simulink model "RoboticFish_Maneuverability_model"  (R2022b)
settings: Solver=ode4  StartTime=0.0  StopTime=50  FixedStep=0.01  RelTol=1e-3  EnableMultiTasking=on
libraries: sharedutil x15, matrix_library x1, dspvision x1, vrlib x1
(part 2 of 3)

== system RoboticFish_Maneuverability_model/Robotic-Fish Model & PropulsionSystem/RF Dynamics and Kinematics (Attitude rappresentation: Quaternions)/6 DOF transformation ==
  note: p q r
  note: u v w
  note: e=[eta;e1;e2;e3]
  note: eta1dot
  note: eta2dot
  eta_E : Inport
  nu : Inport  Port=2
  E1(e) : Subsystem
  E2(e) : Subsystem
  Mux : Mux  Inputs=2
  Product : Product  Inputs=**  Multiplication=Matrix(*)  SaturateOnIntegerOverflow=on  OutDataTypeStr=Inherit: Same as first input
  Product1 : Product  Inputs=**  Multiplication=Matrix(*)  SaturateOnIntegerOverflow=on  OutDataTypeStr=Inherit: Same as first input
  Selector : Selector  InputPortWidth=7  IndexOptions=Index vector (dialog)  Indices=[4 5 6 7]  OutputSizes=1
  Selector1 : Selector  InputPortWidth=6  IndexOptions=Index vector (dialog)  Indices=[1 2 3]  OutputSizes=1
  Selector2 : Selector  InputPortWidth=6  IndexOptions=Index vector (dialog)  Indices=[4 5 6]  OutputSizes=1
  etadot = J(eta_E)*nu : Outport  VectorParamsAs1DForOutWhenUnconnected=off
  E1 : Outport  Port=2  VectorParamsAs1DForOutWhenUnconnected=off
  wires:
  Product1/1 -> Mux/2
  Mux/1 -> etadot = J(eta_E)*nu/1
  Product/1 -> Mux/1
  E2(e)/1(E2) -> Product1/1
  Selector2/1 -> Product1/2
  Selector1/1 -> Product/2
  nu/1 -> Selector2/1, Selector1/1
  E1(e)/1(E1) -> Product/1, E1/1
  eta_E/1 -> Selector/1
  Selector/1 -> E1(e)/1(e), E2(e)/1(e)

== system RoboticFish_Maneuverability_model/Robotic-Fish Model & PropulsionSystem/RF Dynamics and Kinematics (Attitude rappresentation: Quaternions)/Added Mass Coriolis and centripetal matrix ==
  nu_r_B : Inport
  Gain1 : Gain  Gain=-1  SaturateOnIntegerOverflow=on  OutDataTypeStr=Inherit: Same as input  ParamDataTypeStr=Inherit: Same as input
  Gain2 : Gain  Gain=-1  SaturateOnIntegerOverflow=on  OutDataTypeStr=Inherit: Same as input  ParamDataTypeStr=Inherit: Same as input
  M11 : Constant  Value=M11
  M12 : Constant  Value=M12
  M21 : Constant  Value=M21
  M22 : Constant  Value=M22
  Matrix Concatenation : Concatenate  Mode=Multidimensional array
  Matrix Concatenation1 : Concatenate  Mode=Multidimensional array
  Matrix Concatenation2 : Concatenate  Mode=Multidimensional array  ConcatenateDimension=2
  Matrix Multiply{1..4} (4 alike) : Product  Multiplication=Matrix(*)
  Selector1 : Selector  InputPortWidth=6  IndexOptions=Index vector (dialog)  Indices=[1 2 3]  OutputSizes=1
  Selector2 : Selector  InputPortWidth=6  IndexOptions=Index vector (dialog)  Indices=[4 5 6]  OutputSizes=1
  Skew Symmetrical Operator : Subsystem
  "Skew Symmetrical Operator " : Subsystem
  Sum2 : Sum  Inputs=|++  SaturateOnIntegerOverflow=on
  Sum3 : Sum  Inputs=|++  SaturateOnIntegerOverflow=on
  Zero matrix (3 x 3) : Constant  Value=zeros(3,3)
  CA : Outport  VectorParamsAs1DForOutWhenUnconnected=off
  wires:
  Zero matrix (3 x 3)/1 -> Matrix Concatenation/1  "CA(1,1)"
  Matrix Concatenation/1 -> Matrix Concatenation2/1
  Matrix Concatenation1/1 -> Matrix Concatenation2/2
  Matrix Multiply2/1 -> Sum2/1  "M11 * nu_r1_B"
  Matrix Multiply1/1 -> Sum2/2  "M12 * nu_r2_B"
  Matrix Multiply3/1 -> Sum3/1  "M21 * nu_r1_B"
  Selector1/1 -> Matrix Multiply2/2, Matrix Multiply3/2  "nu_r1_B"
  Matrix Multiply4/1 -> Sum3/2  "M22 * nu_r2_B"
  Selector2/1 -> Matrix Multiply1/2, Matrix Multiply4/2  "nu_r2_B"
  Sum2/1 -> "Skew Symmetrical Operator "/1(v)
  Sum3/1 -> Skew Symmetrical Operator/1(v)
  "Skew Symmetrical Operator "/1(S(V)) -> Gain1/1
  Skew Symmetrical Operator/1(S(V)) -> Gain2/1
  Gain1/1 -> Matrix Concatenation1/1, Matrix Concatenation/2  "CA(1,2)"
  Gain2/1 -> Matrix Concatenation1/2  "CA(2,2)"
  nu_r_B/1 -> Selector1/1, Selector2/1
  Matrix Concatenation2/1 -> CA/1
  M11/1 -> Matrix Multiply2/1
  M12/1 -> Matrix Multiply1/1
  M21/1 -> Matrix Multiply3/1
  M22/1 -> Matrix Multiply4/1

== system RoboticFish_Maneuverability_model/Robotic-Fish Model & PropulsionSystem/RF Dynamics and Kinematics (Attitude rappresentation: Quaternions)/Damping forces ==
  nu_r_B : Inport
  Abs : Abs
  Create Diagonal Matrix : matrix_library/Create Diagonal Matrix
  Gain : Gain  Gain=-1
  Linear Damping Matrix : Constant  Value=DL
  Matrix Multiply : Product  Multiplication=Matrix(*)
  Product : Product  SaturateOnIntegerOverflow=on  OutDataTypeStr=Inherit: Same as first input
  Quadratic Damping Vector : Constant  Value=dQ
  Reshape1 : Reshape  OutputDimensionality=Column vector (2-D)
  Reshape2 : Reshape  OutputDimensionality=Column vector (2-D)  OutputDimensions=[6,6]
  Sum1 : Sum  Inputs=|++  SaturateOnIntegerOverflow=on
  D * nu_B : Outport  VectorParamsAs1DForOutWhenUnconnected=off
  wires:
  Reshape2/1 -> Product/1
  Reshape1/1 -> Matrix Multiply/2, Abs/1
  nu_r_B/1 -> Reshape1/1
  Linear Damping Matrix/1 -> Sum1/1
  Create Diagonal Matrix/1 -> Sum1/2
  Product/1 -> Create Diagonal Matrix/1
  Abs/1 -> Product/2  "abs(nu_B)"
  Quadratic Damping Vector/1 -> Reshape2/1  "dQ"
  Matrix Multiply/1 -> D * nu_B/1
  Sum1/1 -> Gain/1  "D"
  Gain/1 -> Matrix Multiply/1

== system RoboticFish_Maneuverability_model/Robotic-Fish Model & PropulsionSystem/RF Dynamics and Kinematics (Attitude rappresentation: Quaternions)/Quaternion normalisation ==
  eta_E : Inport
  Mux : Mux  Inputs=2
  Product : Product  Inputs=*/  SaturateOnIntegerOverflow=on  OutDataTypeStr=Inherit: Same as first input
  Reshape : Reshape  OutputDimensionality=Column vector (2-D)
  Selector : Selector  InputPortWidth=7  IndexOptions=Index vector (dialog)  Indices=[1 2 3]  OutputSizes=1
  Selector1 : Selector  InputPortWidth=7  IndexOptions=Index vector (dialog)  Indices=[4 5 6 7]  OutputSizes=1
  norm 1x4 vector : Subsystem
  eta_E (norm) : Outport  VectorParamsAs1DForOutWhenUnconnected=off
  wires:
  eta_E/1 -> Selector1/1, Selector/1  "eta_E"
  Selector1/1 -> norm 1x4 vector/1(Inport), Product/1
  Selector/1 -> Mux/1
  Product/1 -> Mux/2
  Mux/1 -> Reshape/1
  Reshape/1 -> eta_E (norm)/1
  norm 1x4 vector/1(norm) -> Product/2

== system RoboticFish_Maneuverability_model/Robotic-Fish Model & PropulsionSystem/RF Dynamics and Kinematics (Attitude rappresentation: Quaternions)/Restoring forces ==
  eta_E : Inport
  3x3 Cross Product : sharedutil/3x3 Cross Product  aMode=aMode
  3x3 Cross Product1 : sharedutil/3x3 Cross Product  aMode=aMode
  E1(e) : Subsystem
  Gain : Gain  Gain=-1  SaturateOnIntegerOverflow=on  OutDataTypeStr=Inherit: Same as input  ParamDataTypeStr=Inherit: Same as input
  Matrix Multiply : Product  Multiplication=Matrix(*)
  Matrix Multiply1 : Product  Multiplication=Matrix(*)
  Mux : Mux  Inputs=2
  Selector : Selector  InputPortWidth=7  IndexOptions=Index vector (dialog)  Indices=[4 5 6 7]  OutputSizes=1
  Sum1 : Sum  Inputs=|++  SaturateOnIntegerOverflow=on
  Sum2 : Sum  Inputs=|++  SaturateOnIntegerOverflow=on
  Transpose : Math  Operator=transpose  SignedPower=on
  fB_E : Constant  Value=[0;0;-B]
  fG_E : Constant  Value=[0;0;W]
  rB_B : Constant  Value=rB_B
  rG_B : Constant  Value=rG_B
  g(eta_E)_B : Outport  VectorParamsAs1DForOutWhenUnconnected=off
  wires:
  E1(e)/1(E1) -> Transpose/1  "E1(e)"
  Transpose/1 -> Matrix Multiply/1, Matrix Multiply1/1  "E1(e)^T"
  fG_E/1 -> Matrix Multiply/2
  fB_E/1 -> Matrix Multiply1/2
  Matrix Multiply/1 -> Sum1/1, 3x3 Cross Product/2  "fG_B"
  Matrix Multiply1/1 -> Sum1/2, 3x3 Cross Product1/2  "fB_B"
  rG_B/1 -> 3x3 Cross Product/1
  Sum1/1 -> Mux/1  "fG_B + fB_B"
  3x3 Cross Product/1 -> Sum2/1  "rG_B x fG_B"
  3x3 Cross Product1/1 -> Sum2/2  "rG_B x fG_B"
  rB_B/1 -> 3x3 Cross Product1/1
  Sum2/1 -> Mux/2
  Mux/1 -> Gain/1
  Gain/1 -> g(eta_E)_B/1
  Selector/1 -> E1(e)/1(e)  "e"
  eta_E/1 -> Selector/1  "E1(e)"

== system RoboticFish_Maneuverability_model/Robotic-Fish Model & PropulsionSystem/RF Dynamics and Kinematics (Attitude rappresentation: Quaternions)/Rigid-body Coriolis and centripetal matrix ==
  nu_B : Inport
  Gain : Gain  Gain=m  SaturateOnIntegerOverflow=on  OutDataTypeStr=Inherit: Same as input  ParamDataTypeStr=Inherit: Same as input
  Gain1 : Gain  Gain=-m  SaturateOnIntegerOverflow=on  OutDataTypeStr=Inherit: Same as input  ParamDataTypeStr=Inherit: Same as input
  Gain2 : Gain  Gain=-1  SaturateOnIntegerOverflow=on  OutDataTypeStr=Inherit: Same as input  ParamDataTypeStr=Inherit: Same as input
  Inertia Tensor : Constant  Value=Ib
  Matrix Concatenation : Concatenate  Mode=Multidimensional array
  Matrix Concatenation1 : Concatenate  Mode=Multidimensional array
  Matrix Concatenation2 : Concatenate  Mode=Multidimensional array  ConcatenateDimension=2
  Matrix Multiply : Product  Multiplication=Matrix(*)
  Matrix Multiply1 : Product  Multiplication=Matrix(*)
  Matrix Multiply2 : Product  Multiplication=Matrix(*)
  Selector : Selector  InputPortWidth=6  IndexOptions=Index vector (dialog)  Indices=[4 5 6]  OutputSizes=1
  Selector1 : Selector  InputPortWidth=6  IndexOptions=Index vector (dialog)  Indices=[1 2 3]  OutputSizes=1
  "Skew Symmetrical Operator " : Subsystem
  Skew Symmetrical Operator : Subsystem
  "Skew Symmetrical Operator " : Subsystem
  "Skew Symmetrical Operator  " : Subsystem
  Sum1 : Sum  Inputs=|++  SaturateOnIntegerOverflow=on
  Sum2 : Sum  Inputs=|-+  SaturateOnIntegerOverflow=on
  Zero matrix (3 x 3) : Constant  Value=zeros(3,3)
  rG_B : Constant  Value=rG_B
  CRB : Outport  VectorParamsAs1DForOutWhenUnconnected=off
  wires:
  Gain2/1 -> Matrix Concatenation1/2  "CRB(2,2)"
  Gain/1 -> Matrix Concatenation/2  "CRB(2,1)"
  rG_B/1 -> "Skew Symmetrical Operator  "/1(v)  "rG_B"
  "Skew Symmetrical Operator "/1(S(V)) -> Gain2/1  "S(IO * nu2_B)"
  Selector1/1 -> Skew Symmetrical Operator/1(v)  "nu1_B"
  nu_B/1 -> Selector/1, Selector1/1
  Matrix Concatenation2/1 -> CRB/1
  Skew Symmetrical Operator/1(S(V)) -> Sum2/1, Sum1/1  "S(nu1_B)"
  Gain1/1 -> Matrix Concatenation1/1  "CRB(1,2)"
  Zero matrix (3 x 3)/1 -> Matrix Concatenation/1  "CRB(1,1)"
  Matrix Multiply2/1 -> "Skew Symmetrical Operator "/1(v)  "IO * nu2_B"
  Sum2/1 -> Gain/1
  Matrix Concatenation1/1 -> Matrix Concatenation2/2
  Selector/1 -> "Skew Symmetrical Operator "/1(v), Matrix Multiply2/2  "nu2_B"
  Matrix Multiply/1 -> Sum2/2  "S(rG_B) * S(nu2_B)"
  Inertia Tensor/1 -> Matrix Multiply2/1
  Matrix Concatenation/1 -> Matrix Concatenation2/1
  "Skew Symmetrical Operator "/1(S(V)) -> Matrix Multiply/2, Matrix Multiply1/1  "S(nu2_B)"
  Sum1/1 -> Gain1/1
  Matrix Multiply1/1 -> Sum1/2  "S(nu2_B) * S(rG_B)"
  "Skew Symmetrical Operator  "/1(S(V)) -> Matrix Multiply/1, Matrix Multiply1/2  "S(rG_B)"

== system RoboticFish_Maneuverability_model/Robotic-Fish Model & PropulsionSystem/RF Dynamics and Kinematics (Attitude rappresentation: Quaternions)/Subsystem ==
  "Euler Angles " : Inport
  Add : Sum
  Add1 : Sum  Inputs=-+
  Add2 : Sum
  Add3 : Sum  Inputs=+-
  Demux : Demux  Outputs=3
  Demux1 : Demux  Outputs=3
  Gain : Gain  Gain=0.5
  Mux : Mux
  Product{,1..7} (8 alike) : Product  Inputs=3
  Trigonometric Function : Trigonometry
  Trigonometric Function1 : Trigonometry  Operator=cos
  Quaternions : Outport  VectorParamsAs1DForOutWhenUnconnected=off
  wires:
  "Euler Angles "/1 -> Gain/1
  Gain/1 -> Trigonometric Function1/1, Trigonometric Function/1
  Trigonometric Function/1 -> Demux/1
  Demux/1 -> Product7/1, Product4/1, Product3/1, Product/1  "sin(R/2)"
  Demux/2 -> Product7/2, Product5/2, Product2/2, Product/2  "sin(P/2)"
  Demux/3 -> Product6/3, Product4/3, Product2/3, Product/3  "sin(Y/2)"
  Trigonometric Function1/1 -> Demux1/1
  Demux1/2 -> Product4/2, Product3/2, Product1/2, Product6/2  "cos(P/2)"
  Demux1/1 -> Product6/1, Product1/1, Product2/1, Product5/1  "cos(R/2)"
  Demux1/3 -> Product7/3, Product3/3, Product1/3, Product5/3  "cos(Y/2)"
  Product/1 -> Add/1
  Product1/1 -> Add/2
  Product2/1 -> Add1/1
  Product3/1 -> Add1/2
  Product4/1 -> Add2/1
  Product5/1 -> Add2/2
  Product6/1 -> Add3/1
  Product7/1 -> Add3/2
  Mux/1 -> Quaternions/1
  Add1/1 -> Mux/2
  Add/1 -> Mux/1
  Add2/1 -> Mux/3
  Add3/1 -> Mux/4

== system RoboticFish_Maneuverability_model/State Estimates & VR Animation/VR sink/RF Position and Rotation to VR Translation and Rotation ==
  eta_N : Inport
  Orientation to VR Rotation : Subsystem
  Position to VR Translation : Subsystem
  eta1_N=[x,y,z] : Selector  InputPortWidth=7  IndexOptions=Index vector (dialog)  Indices=[1 2 3]  OutputSizes=1
  eta2_N=[q0,q1,q2,q3] : Selector  InputPortWidth=7  IndexOptions=Index vector (dialog)  Indices=[4 5 6 7]  OutputSizes=1
  VR Rotation : Outport  VectorParamsAs1DForOutWhenUnconnected=off
  VR Translation : Outport  Port=2  VectorParamsAs1DForOutWhenUnconnected=off
  wires:
  Position to VR Translation/1(VR Translation) -> VR Translation/1
  Orientation to VR Rotation/1(VR Rotation) -> VR Rotation/1
  eta_N/1 -> eta2_N=[q0,q1,q2,q3]/1, eta1_N=[x,y,z]/1
  eta1_N=[x,y,z]/1 -> Position to VR Translation/1(Position)
  eta2_N=[q0,q1,q2,q3]/1 -> Orientation to VR Rotation/1(Orientation)

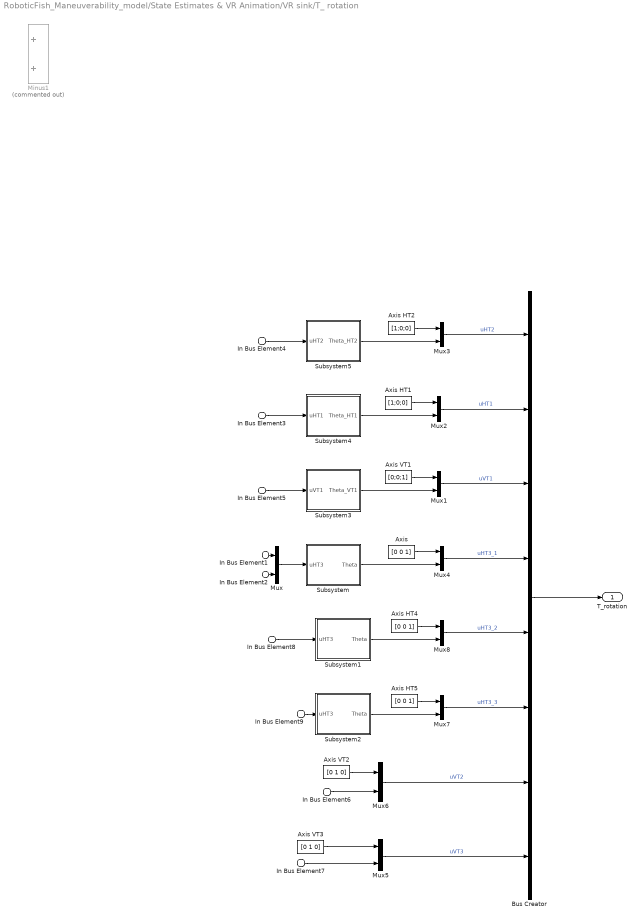
== system RoboticFish_Maneuverability_model/State Estimates & VR Animation/VR sink/T_ rotation ==
  In Bus Element3 : Inport  PortName=uCMD  Element=uHT1
  In Bus Element4 : Inport  PortName=uCMD  Element=uHT2
  In Bus Element5 : Inport  PortName=uCMD  Element=uVT1
  In Bus Element1 : Inport  PortName=uCMD  Element=f_HT3
  In Bus Element8 : Inport  PortName=uCMD  Element=f_HT3
  In Bus Element9 : Inport  PortName=uCMD  Element=f_HT3
  In Bus Element2 : Inport  PortName=uCMD  Element=Thetastr_HT3
  In Bus Element7 : Inport  PortName=uCMD  Element=uVT3
  In Bus Element6 : Inport  PortName=uCMD  Element=uVT2
  Axis : Constant  Value=[0 0 1]
  Axis HT1 : Constant  Value=[1;0;0]
  Axis HT2 : Constant  Value=[1;0;0]
  Axis HT4 : Constant  Value=[0 0 1]
  Axis HT5 : Constant  Value=[0 0 1]
  Axis VT1 : Constant  Value=[0;0;1]
  Axis VT2 : Constant  Value=[0 1 0]
  Axis VT3 : Constant  Value=[0 1 0]
  Bus Creator : BusCreator  Inputs=8
  Minus1 : Sum  Commented=on
  Mux{,1..8} (9 alike) : Mux  Inputs=2
  Subsystem : Subsystem
  Subsystem1 : Subsystem
  Subsystem2 : Subsystem
  Subsystem3 : Subsystem
  Subsystem4 : Subsystem
  Subsystem5 : Subsystem
  T_rotation : Outport  VectorParamsAs1DForOutWhenUnconnected=off
  wires:
  Axis HT1/1 -> Mux2/1
  Bus Creator/1 -> T_rotation/1
  Mux2/1 -> Bus Creator/2  "uHT1"
  Mux3/1 -> Bus Creator/1  "uHT2"
  In Bus Element3/1 -> Subsystem4/1(uHT1)
  Axis HT2/1 -> Mux3/1
  In Bus Element4/1 -> Subsystem5/1(uHT2)
  Subsystem5/1(Theta_HT2) -> Mux3/2
  Subsystem4/1(Theta_HT1) -> Mux2/2
  Subsystem3/1(Theta_VT1) -> Mux1/2
  Mux1/1 -> Bus Creator/3  "uVT1"
  In Bus Element5/1 -> Subsystem3/1(uVT1)
  Axis VT1/1 -> Mux1/1
  In Bus Element2/1 -> Mux/2
  In Bus Element9/1 -> Subsystem2/1(uHT3)
  Mux4/1 -> Bus Creator/4  "uHT3_1"
  Mux7/1 -> Bus Creator/6  "uHT3_3"
  Mux8/1 -> Bus Creator/5  "uHT3_2"
  Mux/1 -> Subsystem/1(uHT3)
  Subsystem2/1(Theta) -> Mux7/2
  Axis HT5/1 -> Mux7/1
  Axis/1 -> Mux4/1
  Axis HT4/1 -> Mux8/1
  In Bus Element1/1 -> Mux/1
  Subsystem1/1(Theta) -> Mux8/2
  Subsystem/1(Theta) -> Mux4/2
  In Bus Element8/1 -> Subsystem1/1(uHT3)
  In Bus Element7/1 -> Mux5/2
  Mux5/1 -> Bus Creator/8  "uVT3"
  Axis VT3/1 -> Mux5/1
  Axis VT2/1 -> Mux6/1
  Mux6/1 -> Bus Creator/7  "uVT2"
  In Bus Element6/1 -> Mux6/2

== system RoboticFish_Maneuverability_model/ALL SCOPE/Subsystem/J1/Subsystem ==
  Roll : Inport
  Constant : Constant
  Constant1 : Constant  Value=0
  Create 3x3 Matrix : sharedutil/Create 3x3 Matrix  aMode=aMode
  Gain : Gain  Gain=-1
  SinCos : Trigonometry  Operator=sincos
  Cx,Roll : Outport
  wires:
  SinCos/1 -> Gain/1, Create 3x3 Matrix/6  "sin(Roll)"
  Constant1/1 -> Create 3x3 Matrix/7, Create 3x3 Matrix/4, Create 3x3 Matrix/3, Create 3x3 Matrix/2
  Gain/1 -> Create 3x3 Matrix/8
  Constant/1 -> Create 3x3 Matrix/1
  SinCos/2 -> Create 3x3 Matrix/9, Create 3x3 Matrix/5  "cos(Roll)"
  Create 3x3 Matrix/1 -> Cx,Roll/1
  Roll/1 -> SinCos/1

== system RoboticFish_Maneuverability_model/ALL SCOPE/Subsystem/J1/Subsystem1 ==
  Pitch : Inport
  Constant : Constant
  Constant1 : Constant  Value=0
  Create 3x3 Matrix : sharedutil/Create 3x3 Matrix  aMode=aMode
  Gain : Gain  Gain=-1
  SinCos : Trigonometry  Operator=sincos
  Cy,Pitch : Outport
  wires:
  SinCos/1 -> Create 3x3 Matrix/7, Gain/1  "sin(Pitch)"
  SinCos/2 -> Create 3x3 Matrix/1, Create 3x3 Matrix/9  "cos(Pitch)"
  Create 3x3 Matrix/1 -> Cy,Pitch/1
  Pitch/1 -> SinCos/1
  Constant1/1 -> Create 3x3 Matrix/8, Create 3x3 Matrix/6, Create 3x3 Matrix/4, Create 3x3 Matrix/2
  Constant/1 -> Create 3x3 Matrix/5
  Gain/1 -> Create 3x3 Matrix/3

== system RoboticFish_Maneuverability_model/ALL SCOPE/Subsystem/J1/Subsystem2 ==
  Yaw : Inport
  Constant : Constant
  Constant1 : Constant  Value=0
  Create 3x3 Matrix : sharedutil/Create 3x3 Matrix  aMode=aMode
  Gain : Gain  Gain=-1
  SinCos : Trigonometry  Operator=sincos
  Cz,Yaw : Outport
  wires:
  Yaw/1 -> SinCos/1
  Create 3x3 Matrix/1 -> Cz,Yaw/1
  SinCos/2 -> Create 3x3 Matrix/5, Create 3x3 Matrix/1  "cos(Yaw)"
  SinCos/1 -> Create 3x3 Matrix/2, Gain/1  "sin(Yaw)"
  Constant1/1 -> Create 3x3 Matrix/8, Create 3x3 Matrix/7, Create 3x3 Matrix/6, Create 3x3 Matrix/3
  Constant/1 -> Create 3x3 Matrix/9
  Gain/1 -> Create 3x3 Matrix/4

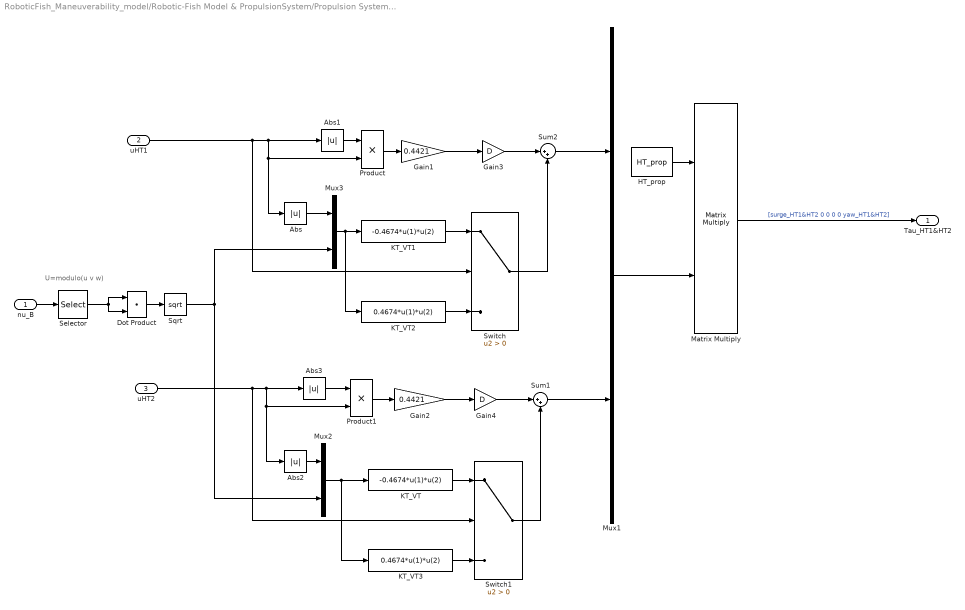
== system RoboticFish_Maneuverability_model/Robotic-Fish Model & PropulsionSystem/Propulsion System/Horizontal Force and Moment (Tau_H)/Tau_HT1&HT2(Tau_Left&Right_Propeller) ==
  note: U=modulo(u v w)
  nu_B : Inport
  uHT1 : Inport  Port=2
  uHT2 : Inport  Port=3
  Abs{,1..3} (4 alike) : Abs  SaturateOnIntegerOverflow=off
  Dot Product : DotProduct  OutDataTypeStr=Inherit: Inherit via internal rule
  Gain1 : Gain  Gain=0.4421
  Gain2 : Gain  Gain=0.4421
  Gain3 : Gain  Gain=D
  Gain4 : Gain  Gain=D
  HT_prop : Constant  Value=HT_prop
  KT_VT : Fcn  Expr=-0.4674*u(1)*u(2)
  KT_VT1 : Fcn  Expr=-0.4674*u(1)*u(2)
  KT_VT2 : Fcn  Expr=0.4674*u(1)*u(2)
  KT_VT3 : Fcn  Expr=0.4674*u(1)*u(2)
  Matrix Multiply : Product  Multiplication=Matrix(*)
  Mux1 : Mux  Inputs=2
  Mux2 : Mux  Inputs=2
  Mux3 : Mux  Inputs=2
  Product : Product
  Product1 : Product
  Selector : Selector  InputPortWidth=6  IndexOptions=Index vector (dialog)  Indices=[1 2 3]  OutputSizes=1
  Sqrt : Sqrt
  Sum1 : Sum  Inputs=|++
  Sum2 : Sum  Inputs=|++
  Switch : Switch  Criteria=u2 > Threshold  SaturateOnIntegerOverflow=off  InputSameDT=off
  Switch1 : Switch  Criteria=u2 > Threshold  SaturateOnIntegerOverflow=off  InputSameDT=off
  Tau_HT1&HT2 : Outport
  wires:
  Product1/1 -> Gain2/1
  Product/1 -> Gain1/1
  Gain1/1 -> Gain3/1
  uHT2/1 -> Switch1/2, Product1/2, Abs2/1, Abs3/1
  HT_prop/1 -> Matrix Multiply/1
  Mux1/1 -> Matrix Multiply/2
  Gain2/1 -> Gain4/1
  Mux2/1 -> KT_VT3/1, KT_VT/1
  Switch1/1 -> Sum1/2
  Matrix Multiply/1 -> Tau_HT1&HT2/1  "[surge_HT1&HT2 0 0 0 0 yaw_HT1&HT2]"
  Sum2/1 -> Mux1/1
  Sum1/1 -> Mux1/2
  KT_VT1/1 -> Switch/1
  Gain3/1 -> Sum2/1
  Gain4/1 -> Sum1/1
  Sqrt/1 -> Mux2/2, Mux3/2
  nu_B/1 -> Selector/1
  Dot Product/1 -> Sqrt/1
  Selector/1 -> Dot Product/2, Dot Product/1
  KT_VT2/1 -> Switch/3
  Mux3/1 -> KT_VT2/1, KT_VT1/1
  Switch/1 -> Sum2/2
  KT_VT/1 -> Switch1/1
  KT_VT3/1 -> Switch1/3
  uHT1/1 -> Switch/2, Abs1/1, Product/2, Abs/1
  Abs1/1 -> Product/1
  Abs/1 -> Mux3/1
  Abs2/1 -> Mux2/1
  Abs3/1 -> Product1/1

== system RoboticFish_Maneuverability_model/Robotic-Fish Model & PropulsionSystem/Propulsion System/Horizontal Force and Moment (Tau_H)/Tau_HT3 (Tau_Caudal_Fin) ==
  "[U uHT3 t]" : Inport
  Bus Creator : BusCreator  Inputs=6
  Calculation_Tau_HT3 : Subsystem
  Constant3 : Constant  Value=[0;0;0;0;0;0]
  Fsurge : Fcn  Expr=(0.5*rho*S*((a0*u(1)^2+a1*u(1)*u(2)*Amp)+a2*(u(2)*Amp)^2)+(b0*u(1)^2+b1*u(1)*u(2)*Amp+b2*(u(2)*Amp)^2)*sin(4*pi*kw*u(2)*u(3)+phisurge))*(1-exp(-u(3)/0.5))
  Fsway : Fcn  Expr=(0.5*rho*S*(sin(2*pi*kw*u(2)*u(3)+phisway)*c2*(u(2)*Amp)^2)*(1-exp(-u(3)/0.5)))
  Myaw : Fcn  Expr=(0.5*rho*S*(sin(2*pi*kw*u(2)*u(3)+phiyaw)*d2*(u(2)*Amp)^2))*(1-exp(-u(3)/0.5))
  Scope1 : Scope  NumInputPorts=2
  Selector : Selector  InputPortWidth=4  IndexOptions=Index vector (dialog)  Indices=[ 3]  OutputSizes=1
  Selector1 : Selector  InputPortWidth=4  IndexOptions=Index vector (dialog)  Indices=[1 2 4]  OutputSizes=1
  Selector3 : Selector  InputPortWidth=3  IndexOptions=Index vector (dialog)  Indices=[2]  OutputSizes=1
  Selector7 : Selector  InputPortWidth=6  IndexOptions=Index vector (dialog)  Indices=[1]  OutputSizes=1
  Selector9 : Selector  InputPortWidth=6  IndexOptions=Index vector (dialog)  Indices=[6]  OutputSizes=1
  SinCos : Trigonometry  Operator=sincos
  Switch : Switch  Criteria=u2 > Threshold  SaturateOnIntegerOverflow=off  InputSameDT=off
  Tau_HT3 : Outport  VectorParamsAs1DForOutWhenUnconnected=off
  wires:
  Calculation_Tau_HT3/1(Tau_HT3) -> Selector7/1, Selector9/1, Switch/1  "[Tau_surge_HT3 Tau_sway_HT3 0 0 0 Tau_yaw_HT3]"
  Switch/1 -> Tau_HT3/1
  Constant3/1 -> Switch/3
  "[U uHT3 t]"/1 -> Selector/1, Selector1/1
  Selector3/1 -> Switch/2  "f"
  Selector1/1 -> Fsurge/1, Selector3/1, Bus Creator/6, Myaw/1, Fsway/1  "[U f_HT3 t]"
  SinCos/1 -> Bus Creator/1  "sin(Thetastr_HT3)"
  SinCos/2 -> Bus Creator/2  "cos(Thetastr_HT3)"
  Fsurge/1 -> Bus Creator/3  "Fsurge"
  Fsway/1 -> Bus Creator/4  "Fsway"
  Myaw/1 -> Bus Creator/5  "Myaw"
  Bus Creator/1 -> Calculation_Tau_HT3/1(InBus)
  Selector/1 -> SinCos/1
  Selector7/1 -> Scope1/1  "Tau_surge_HT3"
  Selector9/1 -> Scope1/2  "Tau_yaw_HT3"

== system RoboticFish_Maneuverability_model/Robotic-Fish Model & PropulsionSystem/Propulsion System/Vertical Force and Moment (Tau_V)/Tau_VT1 (Tau_Middle_Propeller) ==
  note: U=modulo(u v w)
  nu_B : Inport
  uVT1 : Inport  Port=2
  Abs : Abs  SaturateOnIntegerOverflow=off
  Abs1 : Abs  SaturateOnIntegerOverflow=off
  Constant : Constant  Value=VT_prop
  Dot Product : DotProduct  OutDataTypeStr=Inherit: Inherit via internal rule
  Gain : Gain  Gain=0.4421
  Gain3 : Gain  Gain=D
  KT_VT : Fcn  Expr=-0.4674*u(1)*u(2)
  KT_VT1 : Fcn  Expr=0.4674*u(1)*u(2)
  Matrix Multiply : Product  Multiplication=Matrix(*)
  Mux : Mux  Inputs=2
  Product : Product
  Selector : Selector  InputPortWidth=6  IndexOptions=Index vector (dialog)  Indices=[1 2 3]  OutputSizes=1
  Sqrt : Sqrt
  Sum1 : Sum  Inputs=|++
  Switch : Switch  Criteria=u2 > Threshold  SaturateOnIntegerOverflow=off  InputSameDT=off
  Tau_VT1 : Outport
  wires:
  Mux/1 -> KT_VT1/1, KT_VT/1
  Constant/1 -> Matrix Multiply/1
  Product/1 -> Gain/1
  Gain/1 -> Gain3/1
  Matrix Multiply/1 -> Tau_VT1/1
  Sum1/1 -> Matrix Multiply/2
  Gain3/1 -> Sum1/1
  Abs/1 -> Mux/1
  Abs1/1 -> Product/1
  Dot Product/1 -> Sqrt/1
  nu_B/1 -> Selector/1
  Selector/1 -> Dot Product/2, Dot Product/1
  Sqrt/1 -> Mux/2
  KT_VT/1 -> Switch/1
  uVT1/1 -> Abs/1, Abs1/1, Product/2, Switch/2
  KT_VT1/1 -> Switch/3
  Switch/1 -> Sum1/2

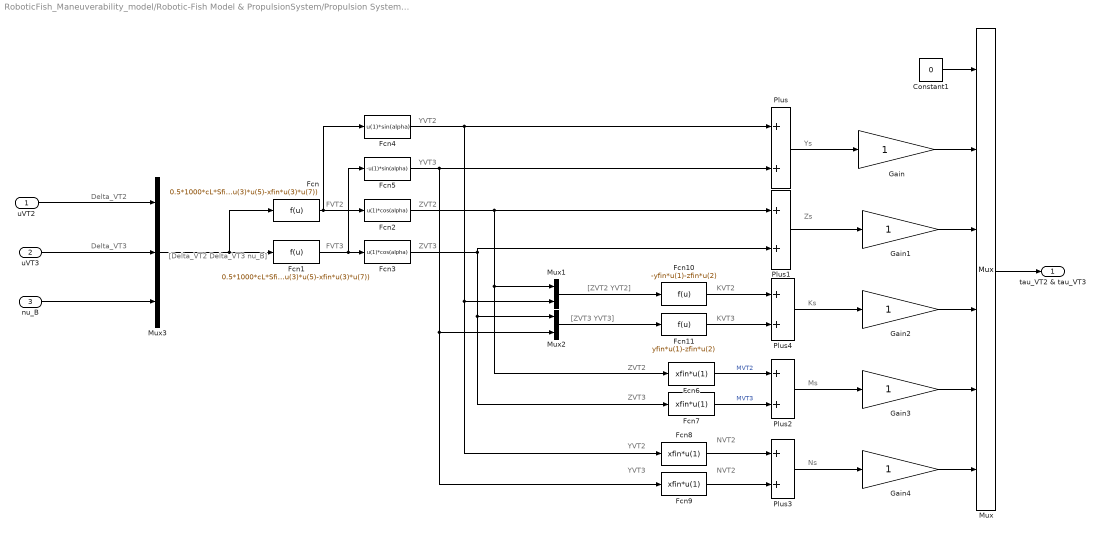
== system RoboticFish_Maneuverability_model/Robotic-Fish Model & PropulsionSystem/Propulsion System/Vertical Force and Moment (Tau_V)/Tau_VT2&VT3 (Tau_Pectoral Fin) ==
  note: Ys
  note: [Delta_VT2 Delta_VT3 nu_B]
  note: Delta_VT2
  note: [ZVT2 YVT2]
  note: FVT2
  note: FVT3
  note: ZVT2
  note: ZVT3
  note: YVT2
  note: YVT3
  note: [ZVT3 YVT3]
  note: KVT3
  note: KVT2
  note: NVT2
  note: NVT2
  note: ZVT3
  note: ZVT2
  note: YVT2
  note: YVT3
  note: Delta_VT3
  note: Zs
  note: Ks
  note: Ms
  note: Ns
  "uVT2 " : Inport
  uVT3 : Inport  Port=2
  nu_B : Inport  Port=3
  Constant1 : Constant  Value=0
  Fcn : Fcn  Expr=0.5*1000*cL*Sfin*(u(3)^2*u(1)+u(3)*u(5)-xfin*u(3)*u(7))
  Fcn1 : Fcn  Expr=0.5*1000*cL*Sfin*(u(3)^2*u(2)+u(3)*u(5)-xfin*u(3)*u(7))
  Fcn10 : Fcn  Expr=-yfin*u(1)-zfin*u(2)
  Fcn11 : Fcn  Expr=yfin*u(1)-zfin*u(2)
  Fcn2 : Fcn  Expr=u(1)*cos(alpha)
  Fcn3 : Fcn  Expr=u(1)*cos(alpha)
  Fcn4 : Fcn  Expr=u(1)*sin(alpha)
  Fcn5 : Fcn  Expr=-u(1)*sin(alpha)
  Fcn{6..9} (4 alike) : Fcn  Expr=xfin*u(1)
  Gain{,1..4} (5 alike) : Gain
  Mux : Mux  Inputs=6
  Mux1 : Mux  Inputs=2
  Mux2 : Mux  Inputs=2
  Mux3 : Mux  Inputs=3
  Plus{,1..4} (5 alike) : Sum
  "tau_VT2 & tau_VT3 " : Outport  VectorParamsAs1DForOutWhenUnconnected=off
  wires:
  Constant1/1 -> Mux/1
  Mux/1 -> "tau_VT2 & tau_VT3 "/1
  Fcn/1 -> Fcn4/1, Fcn2/1
  Fcn1/1 -> Fcn5/1, Fcn3/1
  Fcn4/1 -> Plus/1, Fcn8/1, Mux1/2
  Fcn5/1 -> Fcn9/1, Mux2/2, Plus/2
  Mux1/1 -> Fcn10/1
  Mux2/1 -> Fcn11/1
  Fcn10/1 -> Plus4/1
  Fcn11/1 -> Plus4/2
  Fcn9/1 -> Plus3/2
  Fcn8/1 -> Plus3/1
  Fcn3/1 -> Plus1/2, Fcn7/1, Mux2/1
  Fcn2/1 -> Fcn6/1, Mux1/1, Plus1/1
  Plus/1 -> Gain/1
  Plus4/1 -> Gain2/1
  Plus3/1 -> Gain4/1
  "uVT2 "/1 -> Mux3/1
  uVT3/1 -> Mux3/2
  nu_B/1 -> Mux3/3
  Mux3/1 -> Fcn/1, Fcn1/1
  Gain/1 -> Mux/2
  Gain2/1 -> Mux/4
  Gain4/1 -> Mux/6
  Plus1/1 -> Gain1/1
  Gain1/1 -> Mux/3
  Plus2/1 -> Gain3/1
  Fcn6/1 -> Plus2/1  "MVT2"
  Fcn7/1 -> Plus2/2  "MVT3"
  Gain3/1 -> Mux/5

== system RoboticFish_Maneuverability_model/Robotic-Fish Model & PropulsionSystem/RF Dynamics and Kinematics (Attitude rappresentation: Quaternions)/6 DOF transformation/E1(e) ==
  note: q1,q2,q3
  note: qo
  e : Inport
  Gain : Gain  Gain=2  SaturateOnIntegerOverflow=on  OutDataTypeStr=Inherit: Same as input  ParamDataTypeStr=Inherit: Same as input
  "Gain " : Gain  Gain=2  SaturateOnIntegerOverflow=on  OutDataTypeStr=Inherit: Same as input  ParamDataTypeStr=Inherit: Same as input
  I (3x3) : Constant  Value=eye(3)
  Matrix Multiply : Product  Multiplication=Matrix(*)
  Product : Product  SaturateOnIntegerOverflow=on  OutDataTypeStr=Inherit: Same as first input
  Selector : Selector  InputPortWidth=4  IndexOptions=Index vector (dialog)  Indices=[1]  OutputSizes=1
  Selector1 : Selector  InputPortWidth=4  IndexOptions=Index vector (dialog)  Indices=[2 3 4]  OutputSizes=1
  Skew Symmetrical Operator : Subsystem
  Sum : Sum  Inputs=+++  SaturateOnIntegerOverflow=on
  E1 : Outport  VectorParamsAs1DForOutWhenUnconnected=off
  wires:
  e/1 -> Selector/1, Selector1/1
  Selector/1 -> "Gain "/1  "eta"
  Selector1/1 -> Skew Symmetrical Operator/1(v)  "eps"
  Skew Symmetrical Operator/1(S(V)) -> Matrix Multiply/1, Matrix Multiply/2, Product/2
  Matrix Multiply/1 -> Gain/1
  "Gain "/1 -> Product/1
  I (3x3)/1 -> Sum/1
  Product/1 -> Sum/2
  Gain/1 -> Sum/3
  Sum/1 -> E1/1

== system RoboticFish_Maneuverability_model/Robotic-Fish Model & PropulsionSystem/RF Dynamics and Kinematics (Attitude rappresentation: Quaternions)/6 DOF transformation/E2(e) ==
  note: q=(q1,q2,q3)
  note: q0
  note: 如果将串联维度参数设置为 1，且输入是二维矩阵，模块将执行垂直矩阵串联，并将输入矩阵上下堆叠以创建输出矩阵。
  e : Inport
  Gain : Gain  Gain=0.5  SaturateOnIntegerOverflow=on  OutDataTypeStr=Inherit: Same as input  ParamDataTypeStr=Inherit: Same as input
  Gain1 : Gain  Gain=-1  SaturateOnIntegerOverflow=on  OutDataTypeStr=Inherit: Same as input  ParamDataTypeStr=Inherit: Same as input
  I (3x3) : Constant  Value=eye(3)
  Matrix Concatenation : Concatenate  Mode=Multidimensional array
  Product : Product  SaturateOnIntegerOverflow=on  OutDataTypeStr=Inherit: Same as first input
  Selector : Selector  InputPortWidth=4  IndexOptions=Index vector (dialog)  Indices=[1]  OutputSizes=1
  Selector1 : Selector  InputPortWidth=4  IndexOptions=Index vector (dialog)  Indices=[2 3 4]  OutputSizes=1
  Skew Symmetrical Operator : Subsystem
  Sum : Sum  SaturateOnIntegerOverflow=on
  Transpose : Math  Operator=transpose  SignedPower=on
  E2 : Outport  VectorParamsAs1DForOutWhenUnconnected=off
  wires:
  Selector1/1 -> Skew Symmetrical Operator/1(v), Transpose/1  "eps"
  Selector/1 -> Product/2  "eta"
  e/1 -> Selector1/1, Selector/1
  I (3x3)/1 -> Product/1
  Product/1 -> Sum/1  "eta*I"
  Skew Symmetrical Operator/1(S(V)) -> Sum/2  "S(eps)"
  Transpose/1 -> Gain1/1
  Gain1/1 -> Matrix Concatenation/1  "-eps^T"
  Sum/1 -> Matrix Concatenation/2
  Matrix Concatenation/1 -> Gain/1
  Gain/1 -> E2/1

== system RoboticFish_Maneuverability_model/Robotic-Fish Model & PropulsionSystem/RF Dynamics and Kinematics (Attitude rappresentation: Quaternions)/Added Mass Coriolis and centripetal matrix/Skew Symmetrical Operator ==
  v : Inport
  Constant : Constant  Value=0
  Create 3x3 Matrix : sharedutil/Create 3x3 Matrix  aMode=aMode
  Demux : Demux  Outputs=3
      settings: DisplayOption=none
  Gain : Gain  Gain=-1  SaturateOnIntegerOverflow=on  OutDataTypeStr=Inherit: Same as input  ParamDataTypeStr=Inherit: Same as input
  Gain1 : Gain  Gain=-1  SaturateOnIntegerOverflow=on  OutDataTypeStr=Inherit: Same as input  ParamDataTypeStr=Inherit: Same as input
  Gain2 : Gain  Gain=-1  SaturateOnIntegerOverflow=on  OutDataTypeStr=Inherit: Same as input  ParamDataTypeStr=Inherit: Same as input
  S(V) : Outport  VectorParamsAs1DForOutWhenUnconnected=off
  wires:
  v/1 -> Demux/1
  Create 3x3 Matrix/1 -> S(V)/1
  Gain2/1 -> Create 3x3 Matrix/2  "-v(3)"
  Gain1/1 -> Create 3x3 Matrix/7  "-v(2)"
  Gain/1 -> Create 3x3 Matrix/6  "-v(1)"
  Demux/3 -> Create 3x3 Matrix/4, Gain2/1  "v(3)"
  Demux/2 -> Create 3x3 Matrix/3, Gain1/1  "v(2)"
  Demux/1 -> Create 3x3 Matrix/8, Gain/1  "v(1)"
  Constant/1 -> Create 3x3 Matrix/5, Create 3x3 Matrix/9, Create 3x3 Matrix/1

== system RoboticFish_Maneuverability_model/Robotic-Fish Model & PropulsionSystem/RF Dynamics and Kinematics (Attitude rappresentation: Quaternions)/Added Mass Coriolis and centripetal matrix/Skew Symmetrical Operator  ==
  v : Inport
  Constant : Constant  Value=0
  Create 3x3 Matrix : sharedutil/Create 3x3 Matrix  aMode=aMode
  Demux : Demux  Outputs=3
      settings: DisplayOption=none
  Gain : Gain  Gain=-1  SaturateOnIntegerOverflow=on  OutDataTypeStr=Inherit: Same as input  ParamDataTypeStr=Inherit: Same as input
  Gain1 : Gain  Gain=-1  SaturateOnIntegerOverflow=on  OutDataTypeStr=Inherit: Same as input  ParamDataTypeStr=Inherit: Same as input
  Gain2 : Gain  Gain=-1  SaturateOnIntegerOverflow=on  OutDataTypeStr=Inherit: Same as input  ParamDataTypeStr=Inherit: Same as input
  S(V) : Outport  VectorParamsAs1DForOutWhenUnconnected=off
  wires:
  Constant/1 -> Create 3x3 Matrix/1, Create 3x3 Matrix/9, Create 3x3 Matrix/5
  Demux/1 -> Gain/1, Create 3x3 Matrix/8  "v(1)"
  Demux/2 -> Gain1/1, Create 3x3 Matrix/3  "v(2)"
  Demux/3 -> Gain2/1, Create 3x3 Matrix/4  "v(3)"
  Gain/1 -> Create 3x3 Matrix/6  "-v(1)"
  Gain1/1 -> Create 3x3 Matrix/7  "-v(2)"
  Gain2/1 -> Create 3x3 Matrix/2  "-v(3)"
  Create 3x3 Matrix/1 -> S(V)/1
  v/1 -> Demux/1

== system RoboticFish_Maneuverability_model/Robotic-Fish Model & PropulsionSystem/RF Dynamics and Kinematics (Attitude rappresentation: Quaternions)/Quaternion normalisation/norm 1x4 vector ==
  Inport : Inport
  Plus : Sum  Inputs=++++
  Selector : Selector  InputPortWidth=4  IndexOptions=Index vector (dialog)  Indices=[1]  OutputSizes=1
  Selector1 : Selector  InputPortWidth=4  IndexOptions=Index vector (dialog)  Indices=[2]  OutputSizes=1
  Selector2 : Selector  InputPortWidth=4  IndexOptions=Index vector (dialog)  Indices=[3]  OutputSizes=1
  Selector3 : Selector  InputPortWidth=4  IndexOptions=Index vector (dialog)  Indices=[4]  OutputSizes=1
  Sqrt : Sqrt
  Square{,1..3} (4 alike) : Math  Operator=square  SignedPower=on
  norm : Outport  VectorParamsAs1DForOutWhenUnconnected=off
  wires:
  Square2/1 -> Plus/3
  Square1/1 -> Plus/2
  Square/1 -> Plus/1
  Inport/1 -> Selector3/1, Selector2/1, Selector/1, Selector1/1
  Square3/1 -> Plus/4
  Selector3/1 -> Square3/1
  Plus/1 -> Sqrt/1
  Selector2/1 -> Square2/1
  Sqrt/1 -> norm/1
  Selector1/1 -> Square1/1
  Selector/1 -> Square/1

== system RoboticFish_Maneuverability_model/Robotic-Fish Model & PropulsionSystem/RF Dynamics and Kinematics (Attitude rappresentation: Quaternions)/Restoring forces/E1(e) ==
  e : Inport
  Gain : Gain  Gain=2  SaturateOnIntegerOverflow=on  OutDataTypeStr=Inherit: Same as input  ParamDataTypeStr=Inherit: Same as input
  "Gain " : Gain  Gain=2  SaturateOnIntegerOverflow=on  OutDataTypeStr=Inherit: Same as input  ParamDataTypeStr=Inherit: Same as input
  I (3x3) : Constant  Value=eye(3)
  Matrix Multiply : Product  Multiplication=Matrix(*)
  Product : Product  SaturateOnIntegerOverflow=on  OutDataTypeStr=Inherit: Same as first input
  Selector : Selector  InputPortWidth=4  IndexOptions=Index vector (dialog)  Indices=[1]  OutputSizes=1
  Selector1 : Selector  InputPortWidth=4  IndexOptions=Index vector (dialog)  Indices=[2 3 4]  OutputSizes=1
  Skew Symmetrical Operator : Subsystem
  Sum : Sum  Inputs=+++  SaturateOnIntegerOverflow=on
  E1 : Outport  VectorParamsAs1DForOutWhenUnconnected=off
  wires:
  Sum/1 -> E1/1
  Gain/1 -> Sum/3
  Product/1 -> Sum/2
  I (3x3)/1 -> Sum/1
  "Gain "/1 -> Product/1
  Matrix Multiply/1 -> Gain/1
  Skew Symmetrical Operator/1(S(V)) -> Product/2, Matrix Multiply/2, Matrix Multiply/1
  Selector1/1 -> Skew Symmetrical Operator/1(v)  "eps"
  Selector/1 -> "Gain "/1  "eta"
  e/1 -> Selector1/1, Selector/1

== system RoboticFish_Maneuverability_model/Robotic-Fish Model & PropulsionSystem/RF Dynamics and Kinematics (Attitude rappresentation: Quaternions)/Rigid-body Coriolis and centripetal matrix/Skew Symmetrical Operator  ==
  v : Inport
  Constant : Constant  Value=0
  Create 3x3 Matrix : sharedutil/Create 3x3 Matrix  aMode=aMode
  Demux : Demux  Outputs=3
      settings: DisplayOption=none
  Gain : Gain  Gain=-1  SaturateOnIntegerOverflow=on  OutDataTypeStr=Inherit: Same as input  ParamDataTypeStr=Inherit: Same as input
  Gain1 : Gain  Gain=-1  SaturateOnIntegerOverflow=on  OutDataTypeStr=Inherit: Same as input  ParamDataTypeStr=Inherit: Same as input
  Gain2 : Gain  Gain=-1  SaturateOnIntegerOverflow=on  OutDataTypeStr=Inherit: Same as input  ParamDataTypeStr=Inherit: Same as input
  S(V) : Outport  VectorParamsAs1DForOutWhenUnconnected=off
  wires:
  Constant/1 -> Create 3x3 Matrix/1, Create 3x3 Matrix/9, Create 3x3 Matrix/5
  Demux/1 -> Gain/1, Create 3x3 Matrix/8  "v(1)"
  Demux/2 -> Gain1/1, Create 3x3 Matrix/3  "v(2)"
  Demux/3 -> Gain2/1, Create 3x3 Matrix/4  "v(3)"
  Gain/1 -> Create 3x3 Matrix/6  "-v(1)"
  Gain1/1 -> Create 3x3 Matrix/7  "-v(2)"
  Gain2/1 -> Create 3x3 Matrix/2  "-v(3)"
  Create 3x3 Matrix/1 -> S(V)/1
  v/1 -> Demux/1

== system RoboticFish_Maneuverability_model/Robotic-Fish Model & PropulsionSystem/RF Dynamics and Kinematics (Attitude rappresentation: Quaternions)/Rigid-body Coriolis and centripetal matrix/Skew Symmetrical Operator ==
  v : Inport
  Constant : Constant  Value=0
  Create 3x3 Matrix : sharedutil/Create 3x3 Matrix  aMode=aMode
  Demux : Demux  Outputs=3
      settings: DisplayOption=none
  Gain : Gain  Gain=-1  SaturateOnIntegerOverflow=on  OutDataTypeStr=Inherit: Same as input  ParamDataTypeStr=Inherit: Same as input
  Gain1 : Gain  Gain=-1  SaturateOnIntegerOverflow=on  OutDataTypeStr=Inherit: Same as input  ParamDataTypeStr=Inherit: Same as input
  Gain2 : Gain  Gain=-1  SaturateOnIntegerOverflow=on  OutDataTypeStr=Inherit: Same as input  ParamDataTypeStr=Inherit: Same as input
  S(V) : Outport  VectorParamsAs1DForOutWhenUnconnected=off
  wires:
  Constant/1 -> Create 3x3 Matrix/1, Create 3x3 Matrix/9, Create 3x3 Matrix/5
  Demux/1 -> Gain/1, Create 3x3 Matrix/8  "v(1)"
  Demux/2 -> Gain1/1, Create 3x3 Matrix/3  "v(2)"
  Demux/3 -> Gain2/1, Create 3x3 Matrix/4  "v(3)"
  Gain/1 -> Create 3x3 Matrix/6  "-v(1)"
  Gain1/1 -> Create 3x3 Matrix/7  "-v(2)"
  Gain2/1 -> Create 3x3 Matrix/2  "-v(3)"
  Create 3x3 Matrix/1 -> S(V)/1
  v/1 -> Demux/1

== system RoboticFish_Maneuverability_model/Robotic-Fish Model & PropulsionSystem/RF Dynamics and Kinematics (Attitude rappresentation: Quaternions)/Rigid-body Coriolis and centripetal matrix/Skew Symmetrical Operator  ==
  v : Inport
  Constant : Constant  Value=0
  Create 3x3 Matrix : sharedutil/Create 3x3 Matrix  aMode=aMode
  Demux : Demux  Outputs=3
      settings: DisplayOption=none
  Gain : Gain  Gain=-1  SaturateOnIntegerOverflow=on  OutDataTypeStr=Inherit: Same as input  ParamDataTypeStr=Inherit: Same as input
  Gain1 : Gain  Gain=-1  SaturateOnIntegerOverflow=on  OutDataTypeStr=Inherit: Same as input  ParamDataTypeStr=Inherit: Same as input
  Gain2 : Gain  Gain=-1  SaturateOnIntegerOverflow=on  OutDataTypeStr=Inherit: Same as input  ParamDataTypeStr=Inherit: Same as input
  S(V) : Outport  VectorParamsAs1DForOutWhenUnconnected=off
  wires:
  v/1 -> Demux/1
  Create 3x3 Matrix/1 -> S(V)/1
  Gain2/1 -> Create 3x3 Matrix/2  "-v(3)"
  Gain1/1 -> Create 3x3 Matrix/7  "-v(2)"
  Gain/1 -> Create 3x3 Matrix/6  "-v(1)"
  Demux/3 -> Create 3x3 Matrix/4, Gain2/1  "v(3)"
  Demux/2 -> Create 3x3 Matrix/3, Gain1/1  "v(2)"
  Demux/1 -> Create 3x3 Matrix/8, Gain/1  "v(1)"
  Constant/1 -> Create 3x3 Matrix/5, Create 3x3 Matrix/9, Create 3x3 Matrix/1

== system RoboticFish_Maneuverability_model/Robotic-Fish Model & PropulsionSystem/RF Dynamics and Kinematics (Attitude rappresentation: Quaternions)/Rigid-body Coriolis and centripetal matrix/Skew Symmetrical Operator   ==
  v : Inport
  Constant : Constant  Value=0
  Create 3x3 Matrix : sharedutil/Create 3x3 Matrix  aMode=aMode
  Demux : Demux  Outputs=3
      settings: DisplayOption=none
  Gain : Gain  Gain=-1  SaturateOnIntegerOverflow=on  OutDataTypeStr=Inherit: Same as input  ParamDataTypeStr=Inherit: Same as input
  Gain1 : Gain  Gain=-1  SaturateOnIntegerOverflow=on  OutDataTypeStr=Inherit: Same as input  ParamDataTypeStr=Inherit: Same as input
  Gain2 : Gain  Gain=-1  SaturateOnIntegerOverflow=on  OutDataTypeStr=Inherit: Same as input  ParamDataTypeStr=Inherit: Same as input
  S(V) : Outport  VectorParamsAs1DForOutWhenUnconnected=off
  wires:
  Constant/1 -> Create 3x3 Matrix/1, Create 3x3 Matrix/9, Create 3x3 Matrix/5
  Demux/1 -> Gain/1, Create 3x3 Matrix/8  "v(1)"
  Demux/2 -> Gain1/1, Create 3x3 Matrix/3  "v(2)"
  Demux/3 -> Gain2/1, Create 3x3 Matrix/4  "v(3)"
  Gain/1 -> Create 3x3 Matrix/6  "-v(1)"
  Gain1/1 -> Create 3x3 Matrix/7  "-v(2)"
  Gain2/1 -> Create 3x3 Matrix/2  "-v(3)"
  Create 3x3 Matrix/1 -> S(V)/1
  v/1 -> Demux/1

== system RoboticFish_Maneuverability_model/State Estimates & VR Animation/VR sink/RF Position and Rotation to VR Translation and Rotation/Orientation to VR Rotation ==
  Orientation : Inport
  Add : Sum  Inputs=4
  Constant1 : Constant  Value=[0; 0; 0; 0]
  Demux : Demux
  Demux1 : Demux
  Gain : Gain  Gain=2
  Math Function : Math  Operator=square  SignedPower=on
  Math Function1 : Math  Operator=reciprocal  SignedPower=on
  Mux : Mux
  Product1 : Product
  Sqrt : Sqrt
  Switch : Switch  Criteria=u2 > Threshold  SaturateOnIntegerOverflow=off  InputSameDT=off
  Trigonometric Function : Trigonometry  Operator=acos
  VR Rotation : Outport  VectorParamsAs1DForOutWhenUnconnected=off
  wires:
  Demux1/1 -> Trigonometric Function/1  "q0"
  Switch/1 -> Demux1/1
  Mux/1 -> VR Rotation/1
  Gain/1 -> Mux/4
  Trigonometric Function/1 -> Gain/1
  Product1/1 -> Switch/1
  Math Function/1 -> Demux/1
  Demux/1 -> Add/1
  Demux/4 -> Add/4
  Math Function1/1 -> Product1/2
  Sqrt/1 -> Switch/2, Math Function1/1
  Orientation/1 -> Math Function/1, Product1/1
  Demux/3 -> Add/3
  Constant1/1 -> Switch/3
  Demux/2 -> Add/2
  Add/1 -> Sqrt/1
  Demux1/2 -> Mux/1  "q1"
  Demux1/3 -> Mux/2  "q2"
  Demux1/4 -> Mux/3  "q3"

== system RoboticFish_Maneuverability_model/State Estimates & VR Animation/VR sink/RF Position and Rotation to VR Translation and Rotation/Position to VR Translation ==
  Position : Inport
  Demux : Demux  Outputs=3
  Mux : Mux  Inputs=3
  VR Translation : Outport  VectorParamsAs1DForOutWhenUnconnected=off
  wires:
  Mux/1 -> VR Translation/1
  Position/1 -> Demux/1
  Demux/1 -> Mux/1  "x"
  Demux/2 -> Mux/2  "y"
  Demux/3 -> Mux/3  "z"

== system RoboticFish_Maneuverability_model/State Estimates & VR Animation/VR sink/T_ rotation/Subsystem ==
  uHT3 : Inport
  Amplitude : Constant  Value=0.0973
  Clock : Clock
  Constant : Constant  Value=5.76
  Constant1 : Constant  Value=0
  Constant2 : Constant  Value=1.635
  Constant3 : Constant
  Divide : Product  Inputs=***
  Divide1 : Product  Inputs=***
  Gain1 : Gain  Gain=-1
  Gain2 : Gain  Gain=-1/0.2
  Math Function : Math
  Minus1 : Sum
  Plus1 : Sum
  Plus2 : Sum  Inputs=+-
  Selector : Selector  InputPortWidth=2  IndexOptions=Index vector (dialog)  Indices=[1]  OutputSizes=1
  Selector1 : Selector  InputPortWidth=2  IndexOptions=Index vector (dialog)  Indices=[2]  OutputSizes=1
  Sin : Trigonometry
  Switch : Switch  Criteria=u2 > Threshold  SaturateOnIntegerOverflow=off  InputSameDT=off
  Theta : Outport  VectorParamsAs1DForOutWhenUnconnected=off
  wires:
  Constant/1 -> Divide/1
  uHT3/1 -> Selector/1, Selector1/1
  Constant1/1 -> Switch/3
  Divide/1 -> Minus1/1
  Amplitude/1 -> Divide1/2
  Divide1/1 -> Plus1/2
  Minus1/1 -> Sin/1
  Clock/1 -> Gain2/1, Divide/3  "t"
  Plus1/1 -> Switch/1
  Gain1/1 -> Plus1/1
  Selector1/1 -> Gain1/1
  Switch/1 -> Theta/1
  Sin/1 -> Divide1/3
  Constant2/1 -> Minus1/2
  Selector/1 -> Divide/2, Switch/2  "f"
  Gain2/1 -> Math Function/1
  Math Function/1 -> Plus2/2
  Constant3/1 -> Plus2/1
  Plus2/1 -> Divide1/1

== system RoboticFish_Maneuverability_model/State Estimates & VR Animation/VR sink/T_ rotation/Subsystem1 ==
  uHT3 : Inport
  Amplitude : Constant  Value=0.0760
  Clock : Clock
  Constant : Constant  Value=5.76
  Constant1 : Constant  Value=0
  Constant2 : Constant  Value=2.031
  Constant3 : Constant
  Divide : Product  Inputs=***
  Divide1 : Product  Inputs=***
  Gain2 : Gain  Gain=-1/0.2
  Math Function : Math
  Minus1 : Sum
  Plus2 : Sum  Inputs=+-
  Sin : Trigonometry
  Switch : Switch  Criteria=u2 > Threshold  SaturateOnIntegerOverflow=off  InputSameDT=off
  Theta : Outport  VectorParamsAs1DForOutWhenUnconnected=off
  wires:
  Constant/1 -> Divide/1
  Constant1/1 -> Switch/3
  Divide/1 -> Minus1/1
  Amplitude/1 -> Divide1/2
  Divide1/1 -> Switch/1
  Minus1/1 -> Sin/1
  Switch/1 -> Theta/1
  Sin/1 -> Divide1/3
  Constant2/1 -> Minus1/2
  uHT3/1 -> Divide/2, Switch/2  "f"
  Clock/1 -> Gain2/1, Divide/3  "t"
  Plus2/1 -> Divide1/1
  Math Function/1 -> Plus2/2
  Constant3/1 -> Plus2/1
  Gain2/1 -> Math Function/1

== system RoboticFish_Maneuverability_model/State Estimates & VR Animation/VR sink/T_ rotation/Subsystem2 ==
  uHT3 : Inport
  Amplitude : Constant  Value=0.134
  Clock : Clock
  Constant : Constant  Value=5.76
  Constant1 : Constant  Value=0
  Constant2 : Constant  Value=2.356
  Constant3 : Constant
  Divide : Product  Inputs=***
  Divide1 : Product  Inputs=***
  Gain2 : Gain  Gain=-1/0.2
  Math Function : Math
  Minus1 : Sum
  Plus2 : Sum  Inputs=+-
  Sin : Trigonometry
  Switch : Switch  Criteria=u2 > Threshold  SaturateOnIntegerOverflow=off  InputSameDT=off
  Theta : Outport  VectorParamsAs1DForOutWhenUnconnected=off
  wires:
  Constant/1 -> Divide/1
  Constant1/1 -> Switch/3
  Divide/1 -> Minus1/1
  Amplitude/1 -> Divide1/2
  Minus1/1 -> Sin/1
  Divide1/1 -> Switch/1
  Switch/1 -> Theta/1
  Sin/1 -> Divide1/3
  Constant2/1 -> Minus1/2
  uHT3/1 -> Divide/2, Switch/2  "f"
  Clock/1 -> Gain2/1, Divide/3  "t"
  Plus2/1 -> Divide1/1
  Math Function/1 -> Plus2/2
  Constant3/1 -> Plus2/1
  Gain2/1 -> Math Function/1

== system RoboticFish_Maneuverability_model/State Estimates & VR Animation/VR sink/T_ rotation/Subsystem3 ==
  uVT1 : Inport
  Clock : Clock
  Constant : Constant
  Divide : Product  Inputs=***
  Theta_VT1 : Outport  VectorParamsAs1DForOutWhenUnconnected=off
  wires:
  Constant/1 -> Divide/1
  Clock/1 -> Divide/3  "t"
  uVT1/1 -> Divide/2
  Divide/1 -> Theta_VT1/1

== system RoboticFish_Maneuverability_model/State Estimates & VR Animation/VR sink/T_ rotation/Subsystem4 ==
  uHT1 : Inport
  Clock : Clock
  Constant : Constant  Value=2*pi
  Divide : Product  Inputs=***
  Theta_HT1 : Outport  VectorParamsAs1DForOutWhenUnconnected=off
  wires:
  Constant/1 -> Divide/1
  Clock/1 -> Divide/3  "t"
  uHT1/1 -> Divide/2
  Divide/1 -> Theta_HT1/1

== system RoboticFish_Maneuverability_model/State Estimates & VR Animation/VR sink/T_ rotation/Subsystem5 ==
  uHT2 : Inport
  Clock : Clock
  Constant : Constant  Value=2*pi
  Divide : Product  Inputs=***
  Theta_HT2 : Outport  VectorParamsAs1DForOutWhenUnconnected=off
  wires:
  Constant/1 -> Divide/1
  Clock/1 -> Divide/3  "t"
  uHT2/1 -> Divide/2
  Divide/1 -> Theta_HT2/1

== system RoboticFish_Maneuverability_model/Robotic-Fish Model & PropulsionSystem/Propulsion System/Horizontal Force and Moment (Tau_H)/Tau_HT3 (Tau_Caudal_Fin)/Calculation_Tau_HT3 ==
  note: Tau_yaw_HT3
  In Bus Element1 : Inport  PortName=InBus  Element=sin(Thetastr_HT3)
  In Bus Element2 : Inport  PortName=InBus  Element=cos(Thetastr_HT3)
  In Bus Element3 : Inport  PortName=InBus  Element=Fsurge
  In Bus Element4 : Inport  PortName=InBus  Element=Fsway
  In Bus Element5 : Inport  PortName=InBus  Element=Myaw
  Constant : Constant  Value=0
  Divide{,1,5..6} (4 alike) : Product  Inputs=**
  Gain : Gain  Gain=ld
  Minus : Sum  Inputs=-+
  Mux : Mux  Inputs=2
  Mux1 : Mux  Inputs=5
  Plus : Sum  Inputs=+-
  Plus2 : Sum
  Tau_HT3 : Outport  VectorParamsAs1DForOutWhenUnconnected=off
  wires:
  In Bus Element3/1 -> Divide/1, Divide5/1  "Fsurge"
  In Bus Element2/1 -> Divide/2, Divide6/2  "cos(Thetastr_HT3)"
  Divide/1 -> Plus/1  "Fsurge*cos(Theta_HT3)"
  Divide1/1 -> Plus/2  "Fsway*sin(Theta_HT3)"
  In Bus Element4/1 -> Divide1/1, Divide6/1  "Fsway"
  Divide6/1 -> Plus2/1  "Fsway*cos(Theta_HT3)"
  Divide5/1 -> Plus2/2  "Fsurge*sin(Theta_HT3)"
  Plus2/1 -> Gain/1, Mux/2  "Tau_sway_HT3"
  Plus/1 -> Mux/1  "Tau_surge_HT3"
  Mux/1 -> Mux1/1
  Minus/1 -> Mux1/5
  Constant/1 -> Mux1/2, Mux1/3, Mux1/4
  Mux1/1 -> Tau_HT3/1  "[Tau_surge_HT3 Tau_sway_HT3 0 0 0 Tau_yaw_HT3]"
  In Bus Element1/1 -> Divide1/2, Divide5/2  "sin(Thetastr_HT3)"
  Gain/1 -> Minus/1
  In Bus Element5/1 -> Minus/2

== system RoboticFish_Maneuverability_model/Robotic-Fish Model & PropulsionSystem/RF Dynamics and Kinematics (Attitude rappresentation: Quaternions)/6 DOF transformation/E1(e)/Skew Symmetrical Operator ==
  v : Inport
  Constant : Constant  Value=0
  Create 3x3 Matrix : sharedutil/Create 3x3 Matrix  aMode=aMode
  Demux : Demux  Outputs=3
      settings: DisplayOption=none
  Gain : Gain  Gain=-1  SaturateOnIntegerOverflow=on  OutDataTypeStr=Inherit: Same as input  ParamDataTypeStr=Inherit: Same as input
  Gain1 : Gain  Gain=-1  SaturateOnIntegerOverflow=on  OutDataTypeStr=Inherit: Same as input  ParamDataTypeStr=Inherit: Same as input
  Gain2 : Gain  Gain=-1  SaturateOnIntegerOverflow=on  OutDataTypeStr=Inherit: Same as input  ParamDataTypeStr=Inherit: Same as input
  S(V) : Outport  VectorParamsAs1DForOutWhenUnconnected=off
  wires:
  Constant/1 -> Create 3x3 Matrix/1, Create 3x3 Matrix/9, Create 3x3 Matrix/5
  Demux/1 -> Gain/1, Create 3x3 Matrix/8  "v(1)"
  Demux/2 -> Gain1/1, Create 3x3 Matrix/3  "v(2)"
  Demux/3 -> Gain2/1, Create 3x3 Matrix/4  "v(3)"
  Gain/1 -> Create 3x3 Matrix/6  "-v(1)"
  Gain1/1 -> Create 3x3 Matrix/7  "-v(2)"
  Gain2/1 -> Create 3x3 Matrix/2  "-v(3)"
  Create 3x3 Matrix/1 -> S(V)/1
  v/1 -> Demux/1

== system RoboticFish_Maneuverability_model/Robotic-Fish Model & PropulsionSystem/RF Dynamics and Kinematics (Attitude rappresentation: Quaternions)/6 DOF transformation/E2(e)/Skew Symmetrical Operator ==
  v : Inport
  Constant : Constant  Value=0
  Create 3x3 Matrix : sharedutil/Create 3x3 Matrix  aMode=aMode
  Demux : Demux  Outputs=3
      settings: DisplayOption=none
  Gain : Gain  Gain=-1  SaturateOnIntegerOverflow=on  OutDataTypeStr=Inherit: Same as input  ParamDataTypeStr=Inherit: Same as input
  Gain1 : Gain  Gain=-1  SaturateOnIntegerOverflow=on  OutDataTypeStr=Inherit: Same as input  ParamDataTypeStr=Inherit: Same as input
  Gain2 : Gain  Gain=-1  SaturateOnIntegerOverflow=on  OutDataTypeStr=Inherit: Same as input  ParamDataTypeStr=Inherit: Same as input
  S(V) : Outport  VectorParamsAs1DForOutWhenUnconnected=off
  wires:
  v/1 -> Demux/1
  Create 3x3 Matrix/1 -> S(V)/1
  Gain2/1 -> Create 3x3 Matrix/2  "-v(3)"
  Gain1/1 -> Create 3x3 Matrix/7  "-v(2)"
  Gain/1 -> Create 3x3 Matrix/6  "-v(1)"
  Demux/3 -> Create 3x3 Matrix/4, Gain2/1  "v(3)"
  Demux/2 -> Create 3x3 Matrix/3, Gain1/1  "v(2)"
  Demux/1 -> Create 3x3 Matrix/8, Gain/1  "v(1)"
  Constant/1 -> Create 3x3 Matrix/5, Create 3x3 Matrix/9, Create 3x3 Matrix/1

== system RoboticFish_Maneuverability_model/Robotic-Fish Model & PropulsionSystem/RF Dynamics and Kinematics (Attitude rappresentation: Quaternions)/Restoring forces/E1(e)/Skew Symmetrical Operator ==
  v : Inport
  Constant : Constant  Value=0
  Create 3x3 Matrix : sharedutil/Create 3x3 Matrix  aMode=aMode
  Demux : Demux  Outputs=3
      settings: DisplayOption=none
  Gain : Gain  Gain=-1  SaturateOnIntegerOverflow=on  OutDataTypeStr=Inherit: Same as input  ParamDataTypeStr=Inherit: Same as input
  Gain1 : Gain  Gain=-1  SaturateOnIntegerOverflow=on  OutDataTypeStr=Inherit: Same as input  ParamDataTypeStr=Inherit: Same as input
  Gain2 : Gain  Gain=-1  SaturateOnIntegerOverflow=on  OutDataTypeStr=Inherit: Same as input  ParamDataTypeStr=Inherit: Same as input
  S(V) : Outport  VectorParamsAs1DForOutWhenUnconnected=off
  wires:
  v/1 -> Demux/1
  Create 3x3 Matrix/1 -> S(V)/1
  Gain2/1 -> Create 3x3 Matrix/2  "-v(3)"
  Gain1/1 -> Create 3x3 Matrix/7  "-v(2)"
  Gain/1 -> Create 3x3 Matrix/6  "-v(1)"
  Demux/3 -> Create 3x3 Matrix/4, Gain2/1  "v(3)"
  Demux/2 -> Create 3x3 Matrix/3, Gain1/1  "v(2)"
  Demux/1 -> Create 3x3 Matrix/8, Gain/1  "v(1)"
  Constant/1 -> Create 3x3 Matrix/5, Create 3x3 Matrix/9, Create 3x3 Matrix/1

== matlab function RoboticFish_Maneuverability_model/ALL SCOPE/ESO1/fal(e,0.5,h) ==
  data: u input; y output
function y = fcn(u)
%#codegen 非线性函数fal(x,α,d)
x = u(1);
alpha = u(2);
d = u(3);

if abs(x) <= d
    y = x / (d ^ (1 - alpha));
else 
    y = abs(x) ^ alpha * sign(x);
end

== matlab function RoboticFish_Maneuverability_model/ALL SCOPE/ESO/fal(e,0.25,h) ==
  data: u input; y output
function y = fcn(u)
%#codegen 非线性函数fal(x,α,d)
x = u(1);
alpha = u(2);
d = u(3);

if abs(x) <= d
    y = x / (d ^ (1 - alpha));
else 
    y = abs(x) ^ alpha * sign(x);
end
